simulink model "RALFMain"  (R2018b)
settings: Solver=FixedStepAuto  StartTime=0.0  StopTime=inf  FixedStep=0.001  RelTol=1e-3
InitFcn:
  | init
StopFcn:
  | stop
model workspace (MAT data in the model file):
  SL_ROS_VariableLengthArrays_MaxSizes.CommonInfo.ArrayTruncateAction = 'EmitWarning'
  SL_ROS_VariableLengthArrays_MaxSizes.MsgTypeMap = containers.Map
  SL_ROS_VariableLengthArrays_MaxSizes.MsgTypeMap.serialization.keys = {'sensor_msgs/Joy', 'std_msgs/Float32MultiArray', 'std_msgs/Int16MultiArray', 'std_msgs/Int32MultiArray', 'std_msgs/UInt16MultiArray', 'std_msgs/UInt8MultiArray'}
  SL_ROS_VariableLengthArrays_MaxSizes.MsgTypeMap.serialization.values{1}(1).PropertyName = 'Axes'
  SL_ROS_VariableLengthArrays_MaxSizes.MsgTypeMap.serialization.values{1}(1).DataType = 'single'
  SL_ROS_VariableLengthArrays_MaxSizes.MsgTypeMap.serialization.values{1}(1).MaxLength = 8
  SL_ROS_VariableLengthArrays_MaxSizes.MsgTypeMap.serialization.values{1}(2).PropertyName = 'Buttons'
  SL_ROS_VariableLengthArrays_MaxSizes.MsgTypeMap.serialization.values{1}(2).DataType = 'int32'
  SL_ROS_VariableLengthArrays_MaxSizes.MsgTypeMap.serialization.values{1}(2).MaxLength = 15
  SL_ROS_VariableLengthArrays_MaxSizes.MsgTypeMap.serialization.values{2}.PropertyName = 'Data'
  SL_ROS_VariableLengthArrays_MaxSizes.MsgTypeMap.serialization.values{2}.DataType = 'single'
  SL_ROS_VariableLengthArrays_MaxSizes.MsgTypeMap.serialization.values{2}.MaxLength = 8
  SL_ROS_VariableLengthArrays_MaxSizes.MsgTypeMap.serialization.values{3}.PropertyName = 'Data'
  SL_ROS_VariableLengthArrays_MaxSizes.MsgTypeMap.serialization.values{3}.DataType = 'int16'
  SL_ROS_VariableLengthArrays_MaxSizes.MsgTypeMap.serialization.values{3}.MaxLength = 4
  SL_ROS_VariableLengthArrays_MaxSizes.MsgTypeMap.serialization.values{4}.PropertyName = 'Data'
  SL_ROS_VariableLengthArrays_MaxSizes.MsgTypeMap.serialization.values{4}.DataType = 'int32'
  SL_ROS_VariableLengthArrays_MaxSizes.MsgTypeMap.serialization.values{4}.MaxLength = 8
  SL_ROS_VariableLengthArrays_MaxSizes.MsgTypeMap.serialization.values{5}.PropertyName = 'Data'
  SL_ROS_VariableLengthArrays_MaxSizes.MsgTypeMap.serialization.values{5}.DataType = 'uint16'
  SL_ROS_VariableLengthArrays_MaxSizes.MsgTypeMap.serialization.values{5}.MaxLength = 8
  SL_ROS_VariableLengthArrays_MaxSizes.MsgTypeMap.serialization.values{6}.PropertyName = 'Data'
  SL_ROS_VariableLengthArrays_MaxSizes.MsgTypeMap.serialization.values{6}.DataType = 'uint8'
  SL_ROS_VariableLengthArrays_MaxSizes.MsgTypeMap.serialization.values{6}.MaxLength = 8
  SL_ROS_VariableLengthArrays_MaxSizes.MsgTypeMap.serialization.uniformity = 0
  SL_ROS_VariableLengthArrays_MaxSizes.MsgTypeMap.serialization.keyType = 'char'
  SL_ROS_VariableLengthArrays_MaxSizes.MsgTypeMap.serialization.valueType = 'any'
undefined symbols (not defined in the file): Axes, Axes_SL_Info, Buttons, Buttons_SL_Info, kp, nmax, pwinkel, pwinkel_R, pwinkel_vel
libraries: simulink x15, etargetslib x10, cstblocks x4, robotlib x4, dspswit3 x4, simulink_extras x4, robotcorelib x1
CloseFcn:
  | stop
settings Model: EnablePacing=on  Creator=alf  LastModifiedBy=alf
settings OptimizationCC: EnhancedBackFolding=on  PassReuseOutputArgsAs=Individual arguments  MaxStackSize=64  OptimizeBlockOrder=speed  DifferentSizesBufferReuse=on  OptimizationCustomize=off
settings DebuggingCC: ParameterPrecisionLossMsg=none  ParameterTunabilityLossMsg=error
settings HardwareCC: ProdBitPerLong=64  ProdHWDeviceType=Intel->x86-64 (Linux 64)
settings SFSimCC: MATLABDynamicMemAlloc=off
settings RTWCC: SystemTargetFile=ert.tlc  HardwareBoard=Robot Operating System (ROS)  TLCOptions="-aInlineSetEventsForThisBaseRateFcn=TLC_FALSE -aSuppressMultiTaskScheduler=TLC_FALSE  -aRateBasedStepFcn=0"  TemplateMakefile=ert_default_tmf  GenerateReport=on  Toolchain=Catkin  IncludeHyperlinkInReport=on  LaunchReport=on  TargetLang=C++  GenerateTraceInfo=on  GenerateTraceReport=on  GenerateTraceReportSl=on  GenerateTraceReportSf=on  GenerateTraceReportEml=on
settings CodeAppCC: ForceParamTrailComments=on  IgnoreCustomStorageClasses=off  OperatorAnnotations=on  SimulinkDataObjDesc=on  SFDataObjDesc=on  InsertBlockDesc=on
settings ERTTargetCC: SupportContinuousTime=on  SupportNonInlinedSFcns=on

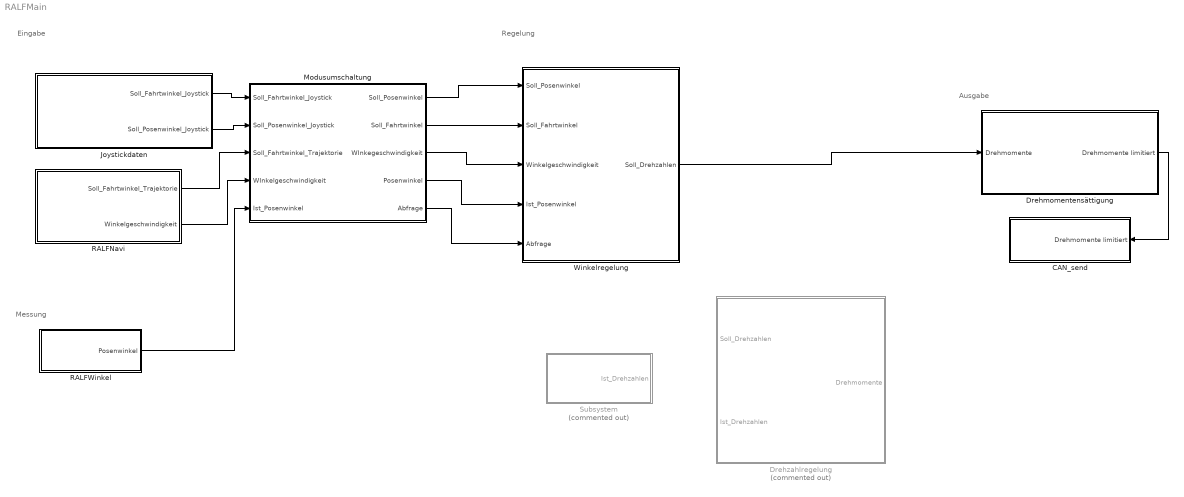
== system RALFMain ==
  note: Ausgabe
  note: Eingabe
  note: Messung
  note: Regelung
  CAN_send : Subsystem
  Drehmomentensättigung : Subsystem
  Drehzahlregelung : Subsystem  Commented=on
  Joystickdaten : Subsystem
  Modusumschaltung : Subsystem
  RALFNavi : Subsystem
  RALFWinkel : Subsystem
  Subsystem : Subsystem  Commented=on
  Winkelregelung : Subsystem
  wires:
  Modusumschaltung/1(Soll_Posenwinkel) -> Winkelregelung/1(Soll_Posenwinkel)
  Modusumschaltung/2(Soll_Fahrtwinkel) -> Winkelregelung/2(Soll_Fahrtwinkel)
  Joystickdaten/1(Soll_Fahrtwinkel_Joystick) -> Modusumschaltung/1(Soll_Fahrtwinkel_Joystick)
  Joystickdaten/2(Soll_Posenwinkel_Joystick) -> Modusumschaltung/2(Soll_Posenwinkel_Joystick)
  Modusumschaltung/4(Posenwinkel) -> Winkelregelung/4(Ist_Posenwinkel)
  Modusumschaltung/3(WInkegeschwindigkeit) -> Winkelregelung/3(Winkelgeschwindigkeit)
  RALFWinkel/1(Posenwinkel) -> Modusumschaltung/5(Ist_Posenwinkel)
  RALFNavi/1(Soll_Fahrtwinkel_Trajektorie) -> Modusumschaltung/3(Soll_Fahrtwinkel_Trajektorie)
  RALFNavi/2("Winkelgeschwindigkeit ") -> Modusumschaltung/4("WInkelgeschwindigkeit ")
  Modusumschaltung/5(Abfrage) -> Winkelregelung/5("Abfrage ")
  Drehmomentensättigung/1(Drehmomente limitiert) -> CAN_send/1(Drehmomente limitiert)
  Winkelregelung/1(Soll_Drehzahlen) -> Drehmomentensättigung/1(Drehmomente)

== system RALFMain/CAN_send ==
  Drehmomente limitiert : Inport
  CAN send back left : S-Function  FunctionName=CAN_send  Parameters=Port,Identifier  SFunctionModules=socketcan  SFunctionDeploymentMode=off  EnableBusSupport=off  mask{Port=can0, Identifier=hex2dec('121')}
      mask prompts: Port "CAN Port"
      mask TypeOptions Port: can0 | can1 | can2
      mask DialogControl DescTextVar Prompt: Dennis Hotze, Dominik Eickmann
  CAN send back right : S-Function  FunctionName=CAN_send  Parameters=Port,Identifier  SFunctionModules=socketcan  SFunctionDeploymentMode=off  EnableBusSupport=off  mask{Port=can0, Identifier=hex2dec('131')}
      mask prompts: Port "CAN Port"
      mask TypeOptions Port: can0 | can1 | can2
      mask DialogControl DescTextVar Prompt: Dennis Hotze, Dominik Eickmann
  CAN send front left : S-Function  FunctionName=CAN_send  Parameters=Port,Identifier  SFunctionModules=socketcan  SFunctionDeploymentMode=off  EnableBusSupport=off  mask{Port=can0, Identifier=hex2dec('111')}
      mask prompts: Port "CAN Port"
      mask TypeOptions Port: can0 | can1 | can2
      mask DialogControl DescTextVar Prompt: Dennis Hotze, Dominik Eickmann
  CAN send front right : S-Function  FunctionName=CAN_send  Parameters=Port,Identifier  SFunctionModules=socketcan  SFunctionDeploymentMode=off  EnableBusSupport=off  mask{Port=can0, Identifier=hex2dec('101')}
      mask prompts: Port "CAN Port"
      mask TypeOptions Port: can0 | can1 | can2
      mask DialogControl DescTextVar Prompt: Dennis Hotze, Dominik Eickmann
  Demux : Demux
  wires:
  Demux/4 -> CAN send back right/1
  Demux/1 -> CAN send front right/1
  Demux/2 -> CAN send front left/1
  Drehmomente limitiert/1 -> Demux/1
  Demux/3 -> CAN send back left/1

== system RALFMain/Drehmomentensättigung ==
  note: Inaktiv
  Drehmomente : Inport
  Abfrage DMS-Betaetigung : Subsystem
  Conversion MiControll : Subsystem
  Product : Product
  Sättigung/Conversion EPOS : Subsystem  Commented=on
  Drehmomente limitiert : Outport
  wires:
  Drehmomente/1 -> Product/1
  Abfrage DMS-Betaetigung/1("DMS-Betaetigung ") -> Product/2
  Product/1 -> Conversion MiControll/1(In1)
  Conversion MiControll/1(Out1) -> Drehmomente limitiert/1

== system RALFMain/Drehzahlregelung ==
  note: Inaktiv
  Soll_Drehzahlen : Inport
  Ist_Drehzahlen : Inport  Port=2
  PID Controller : simulink/Continuous/PID Controller  Controller=PID  Form=Ideal  TimeDomain=Continuous-time  SampleTime=-1  IntegratorMethod=Forward Euler  FilterMethod=Forward Euler  ControllerParametersSource=internal  P=0.05105  I=0.78114  D=0  UseFilter=on  N=100  TunerSelectOption=Transfer Function Based (PID Tuner App)  InitialConditionSource=internal  InitialConditionForIntegrator=0  InitialConditionForFilter=0  DifferentiatorICPrevScaledInput=0  ExternalReset=none  TrackingMode=off  Kt=1  LimitOutput=on  UpperSaturationLimit=inf  LowerSaturationLimit=-inf  LinearizeAsGain=on  AntiWindupMode=back-calculation  Kb=1  POutMin=[]  POutMax=[]  IOutMin=[]  IOutMax=[]  DOutMin=[]  DOutMax=[]  NOutMin=[]  NOutMax=[]  SumOutMin=[]  SumOutMax=[]  SaturationOutMin=[]  SaturationOutMax=[]  PParamMin=[]  PParamMax=[]  IParamMin=[]  IParamMax=[]  DParamMin=[]  DParamMax=[]  NParamMin=[]  NParamMax=[]  KbParamMin=[]  KbParamMax=[]  KtParamMin=[]  KtParamMax=[]  KbOutMin=[]  KbOutMax=[]  KtOutMin=[]  KtOutMax=[]  IntegratorOutMin=[]  IntegratorOutMax=[]  FilterOutMin=[]  FilterOutMax=[]  SumI1OutMin=[]  SumI1OutMax=[]  SumI2OutMin=[]  SumI2OutMax=[]  SumI3OutMin=[]  SumI3OutMax=[]  SumI4OutMin=[]  SumI4OutMax=[]  SumDOutMin=[]  SumDOutMax=[]  DifferentiatorOutMin=[]  DifferentiatorOutMax=[]  FilterDiffOutCoefMin=[]  FilterDiffOutCoefMax=[]  ReciprocalOutMin=[]  ReciprocalOutMax=[]  SumDenOutMin=[]  SumDenOutMax=[]  SumNumOutMin=[]  SumNumOutMax=[]  DivideOutMin=[]  DivideOutMax=[]  IntegratorContinuousStateAttributes=''  IntegratorStateMustResolveToSignalObject=off  IntegratorRTWStateStorageClass=Auto  FilterContinuousStateAttributes=''  FilterStateMustResolveToSignalObject=off  FilterRTWStateStorageClass=Auto  ParallelPVariant=Passthrough  IdealPVariant=InternalParameters  IVariant=InternalParameters  DVariant=InternalParameters  IntegratorVariant=Continuous  SatVariant=Enabled  AWVariant=BackCalculation  PCopyVariant=Disabled  TRVariant=Disabled  FdbkBlocksVariant=Forward  IdealPFdbkVariant=Disabled  SatFdbkVariant=Disabled  DerivativeFilterVariant=ContFilter  NVariant=InternalParameters  NCopyVariant=Disabled  FilterICVariant=InternalICsFilter  IntegratorICVariant=InternalICs  ExternalResetVariant=Disabled  TRSumVariant=Passthrough  SumFdbkVariant=Disabled  SumVariant=Sum_PID
  Regelung RALF : Subsystem  Commented=on
  Sum : Sum  Inputs=|+-
  Drehmomente : Outport
  wires:
  Soll_Drehzahlen/1 -> Sum/1
  Ist_Drehzahlen/1 -> Sum/2
  Sum/1 -> PID Controller/1
  PID Controller/1 -> Drehmomente/1

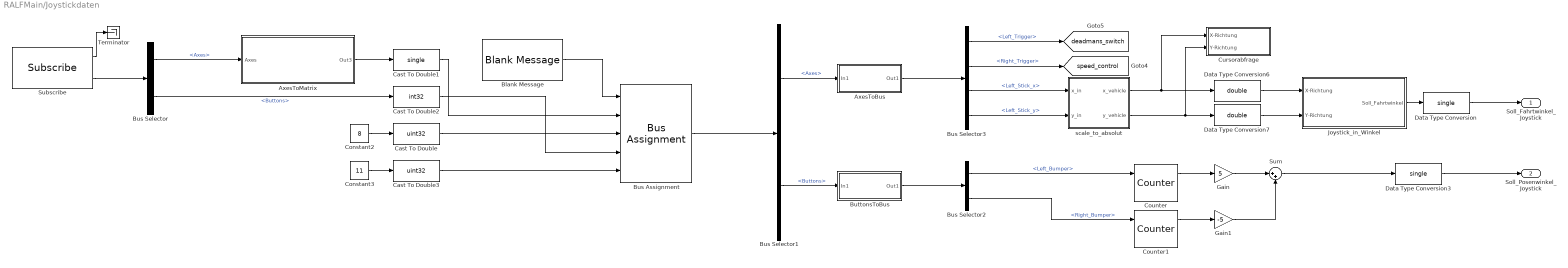
== system RALFMain/Joystickdaten ==
  AxesToBus : Subsystem
  AxesToMatrix : Subsystem
  Blank Message : robotlib/Blank Message  messageClass=Message  entityType=sensor_msgs/Joy  messageType=sensor_msgs/Joy  SampleTime=inf
      settings: SourceProductBaseCode=RO
  Bus Assignment : BusAssignment  AssignedSignals=Axes,Axes_SL_Info.CurrentLength,Buttons,Buttons_SL_Info.CurrentLength
  Bus Selector : BusSelector  OutputSignals=Axes,Buttons
  Bus Selector1 : BusSelector  OutputSignals=Axes,Buttons
  Bus Selector2 : BusSelector  OutputSignals=Bumper.Left_Bumper,Bumper.Right_Bumper
  Bus Selector3 : BusSelector  OutputSignals=Trigger.Left_Trigger,Trigger.Right_Trigger,Left_Stick.Left_Stick_x,Left_Stick.Left_Stick_y
  ButtonsToBus : Subsystem
  Cast To Double : DataTypeConversion  OutDataTypeStr=uint32
  Cast To Double1 : DataTypeConversion  OutDataTypeStr=single
  Cast To Double2 : DataTypeConversion  OutDataTypeStr=int32
  Cast To Double3 : DataTypeConversion  OutDataTypeStr=uint32
  Constant2 : Constant  Value=8
  Constant3 : Constant  Value=11
  Counter : dspswit3/Counter  Direction=Up  CountEvent=Rising edge  CounterSize=User defined  MaxCount=255  InitialCount=0  Output=Count and Hit  HitValue=32  ResetInput=on  SamplesPerFrame=1  Ts=1  CntDtype=double  HitDtype=Logical
  Counter1 : dspswit3/Counter  Direction=Up  CountEvent=Rising edge  CounterSize=User defined  MaxCount=255  InitialCount=0  Output=Count and Hit  HitValue=32  ResetInput=on  SamplesPerFrame=1  Ts=1  CntDtype=double  HitDtype=Logical
  Cursorabfrage : Subsystem
  Data Type Conversion : DataTypeConversion  OutDataTypeStr=single
  Data Type Conversion3 : DataTypeConversion  OutDataTypeStr=single
  Data Type Conversion6 : DataTypeConversion  OutDataTypeStr=double
  Data Type Conversion7 : DataTypeConversion  OutDataTypeStr=double
  Gain : Gain  Gain=5
  Gain1 : Gain  Gain=-5
  Joystick_in_Winkel : Subsystem
  Subscribe : robotlib/Subscribe  topicSource=Select from ROS network  topic=/joy  messageType=sensor_msgs/Joy  sampleTime=-1  messageQueueLength=1
      settings: SourceProductBaseCode=RO
  Sum : Sum  Inputs=|++
  Terminator : Terminator
  scale_to_absolut : Subsystem
  Soll_Fahrtwinkel_Joystick : Outport
  Soll_Posenwinkel_Joystick : Outport  Port=2
  tag scope: deadmans_switch=global, speed_control=global
  wires:
  Bus Selector2/2 -> Counter1/1  "<Right_Bumper>"
  Bus Selector2/1 -> Counter/1  "<Left_Bumper>"
  AxesToBus/1(Out1) -> Bus Selector3/1
  Bus Selector1/1 -> AxesToBus/1(In1)  "<Axes>"
  Bus Selector3/4 -> scale_to_absolut/2(y_in)  "<Left_Stick_y>"
  Bus Assignment/1 -> Bus Selector1/1
  ButtonsToBus/1(Out1) -> Bus Selector2/1
  Bus Selector3/3 -> scale_to_absolut/1(x_in)  "<Left_Stick_x>"
  Bus Selector1/2 -> ButtonsToBus/1(In1)  "<Buttons>"
  Bus Selector3/1 -> [deadmans_switch]  "<Left_Trigger>"
  scale_to_absolut/1(x_vehicle) -> Cursorabfrage/1(X-Richtung), Data Type Conversion6/1
  Data Type Conversion7/1 -> Joystick_in_Winkel/2(Y-Richtung)
  Data Type Conversion6/1 -> Joystick_in_Winkel/1(X-Richtung)
  Data Type Conversion/1 -> Soll_Fahrtwinkel_Joystick/1
  Joystick_in_Winkel/1(Soll_Fahrtwinkel) -> Data Type Conversion/1
  Data Type Conversion3/1 -> Soll_Posenwinkel_Joystick/1
  Sum/1 -> Data Type Conversion3/1
  scale_to_absolut/2(y_vehicle) -> Cursorabfrage/2(Y-Richtung), Data Type Conversion7/1
  Constant3/1 -> Cast To Double3/1
  Cast To Double1/1 -> Bus Assignment/2
  Blank Message/1 -> Bus Assignment/1
  AxesToMatrix/1(Out3) -> Cast To Double1/1
  Bus Selector/2 -> Cast To Double2/1  "<Buttons>"
  Constant2/1 -> Cast To Double/1
  Cast To Double/1 -> Bus Assignment/3
  Subscribe/2 -> Bus Selector/1
  Cast To Double2/1 -> Bus Assignment/4
  Subscribe/1 -> Terminator/1
  Bus Selector/1 -> AxesToMatrix/1(Axes)  "<Axes>"
  Cast To Double3/1 -> Bus Assignment/5
  Bus Selector3/2 -> [speed_control]  "<Right_Trigger>"
  Counter/1 -> Gain/1
  Gain/1 -> Sum/1
  Counter1/1 -> Gain1/1
  Gain1/1 -> Sum/2

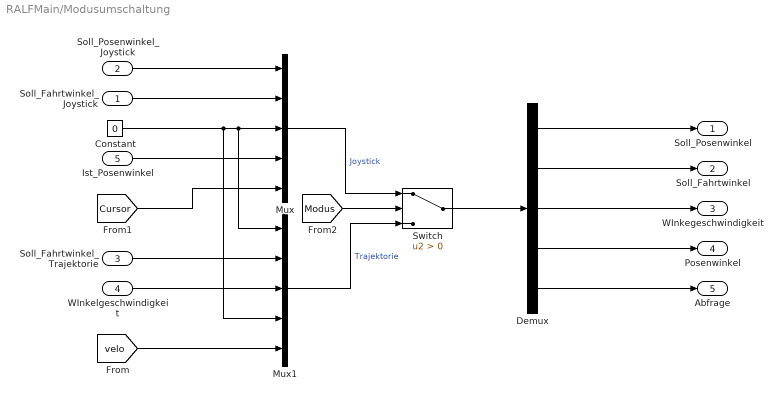
== system RALFMain/Modusumschaltung ==
  Soll_Fahrtwinkel_Joystick : Inport
  Soll_Posenwinkel_Joystick : Inport  Port=2
  Soll_Fahrtwinkel_Trajektorie : Inport  Port=3
  "WInkelgeschwindigkeit " : Inport  Port=4
  Ist_Posenwinkel : Inport  Port=5
  Constant : Constant  Value=0  OutDataTypeStr=single
  Demux : Demux  Outputs=5
  Mux : Mux  Inputs=5
  Mux1 : Mux  Inputs=5
  Switch : Switch  Criteria=u2 > Threshold
  Soll_Posenwinkel : Outport
  Soll_Fahrtwinkel : Outport  Port=2
  WInkegeschwindigkeit : Outport  Port=3
  Posenwinkel : Outport  Port=4
  Abfrage : Outport  Port=5
  wires:
  Switch/1 -> Demux/1
  Demux/2 -> Soll_Fahrtwinkel/1
  Demux/1 -> Soll_Posenwinkel/1
  Soll_Fahrtwinkel_Joystick/1 -> Mux/2
  Mux/1 -> Switch/1  "Joystick"
  Mux1/1 -> Switch/3  "Trajektorie"
  Constant/1 -> Mux1/4, Mux1/1, Mux/3
  Demux/3 -> WInkegeschwindigkeit/1
  Demux/4 -> Posenwinkel/1
  Soll_Posenwinkel_Joystick/1 -> Mux/1
  Ist_Posenwinkel/1 -> Mux/4
  Soll_Fahrtwinkel_Trajektorie/1 -> Mux1/2
  "WInkelgeschwindigkeit "/1 -> Mux1/3
  [Cursor] -> Mux/5
  [velo] -> Mux1/5
  Demux/5 -> Abfrage/1
  [Modus] -> Switch/2

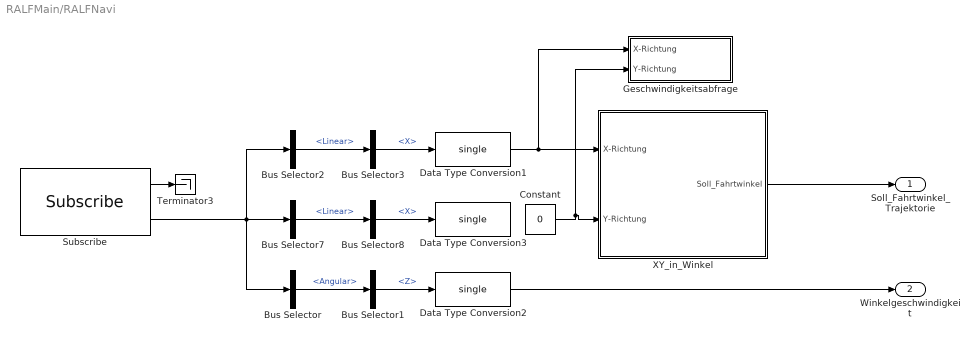
== system RALFMain/RALFNavi ==
  Bus Selector : BusSelector  OutputSignals=Angular
  Bus Selector1 : BusSelector  OutputSignals=Z
  Bus Selector2 : BusSelector  OutputSignals=Linear
  Bus Selector3 : BusSelector  OutputSignals=X
  Bus Selector7 : BusSelector  OutputSignals=Linear
  Bus Selector8 : BusSelector  OutputSignals=X
  Constant : Constant  Value=0  OutDataTypeStr=single
  Data Type Conversion1 : DataTypeConversion  OutDataTypeStr=single
  Data Type Conversion2 : DataTypeConversion  OutDataTypeStr=single
  Data Type Conversion3 : DataTypeConversion  OutDataTypeStr=single
  Geschwindigkeitsabfrage : Subsystem
  Subscribe : robotlib/Subscribe  topicSource=Select from ROS network  topic=/cmd_vel  messageType=geometry_msgs/Twist  sampleTime=-1  messageQueueLength=1
      settings: SourceProductBaseCode=RO
  Terminator3 : Terminator
  XY_in_Winkel : Subsystem
  Soll_Fahrtwinkel_Trajektorie : Outport
  "Winkelgeschwindigkeit " : Outport  Port=2
  wires:
  Bus Selector3/1 -> Data Type Conversion1/1  "<X>"
  Bus Selector2/1 -> Bus Selector3/1  "<Linear>"
  Bus Selector7/1 -> Bus Selector8/1  "<Linear>"
  Data Type Conversion2/1 -> "Winkelgeschwindigkeit "/1
  Bus Selector8/1 -> Data Type Conversion3/1  "<X>"
  Subscribe/2 -> Bus Selector7/1, Bus Selector/1, Bus Selector2/1
  Bus Selector1/1 -> Data Type Conversion2/1  "<Z>"
  Bus Selector/1 -> Bus Selector1/1  "<Angular>"
  Subscribe/1 -> Terminator3/1
  XY_in_Winkel/1(Soll_Fahrtwinkel) -> Soll_Fahrtwinkel_Trajektorie/1
  Data Type Conversion1/1 -> Geschwindigkeitsabfrage/1(X-Richtung), XY_in_Winkel/1(X-Richtung)
  Constant/1 -> Geschwindigkeitsabfrage/2(Y-Richtung), XY_in_Winkel/2(Y-Richtung)

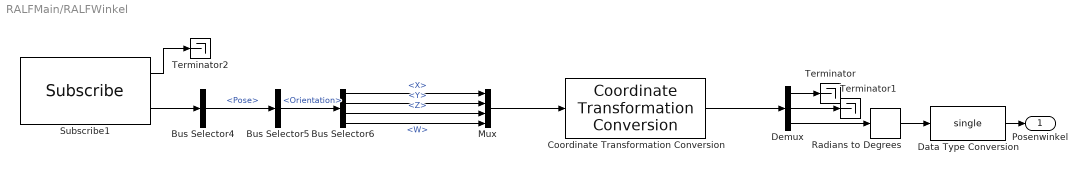
== system RALFMain/RALFWinkel ==
  Bus Selector4 : BusSelector  OutputSignals=Pose
  Bus Selector5 : BusSelector  OutputSignals=Orientation
  Bus Selector6 : BusSelector  OutputSignals=X,Y,Z,W
  Coordinate Transformation Conversion : robotcorelib/Coordinate Transformation Conversion  InputRepresentation=Quaternion  InputEulerSequence=ZYX  ShowTrVecInputPort=on  OutputRepresentation=Euler Angles  OutputEulerSequence=ZYX  ShowTrVecOutputPort=on  SimulateUsing=Interpreted execution
      settings: SourceProductBaseCode=RO
  Data Type Conversion : DataTypeConversion  OutDataTypeStr=single
  Demux : Demux  Outputs=3
  Mux : Mux
  Radians to Degrees : simulink_extras/Transformations/Radians to Degrees
  Subscribe1 : robotlib/Subscribe  topicSource=Select from ROS network  topic=/slam_out_pose  messageType=geometry_msgs/PoseStamped  sampleTime=-1  messageQueueLength=1
      settings: SourceProductBaseCode=RO
  Terminator : Terminator
  Terminator1 : Terminator
  Terminator2 : Terminator
  Posenwinkel : Outport
  wires:
  Bus Selector6/4 -> Mux/4  "<W>"
  Bus Selector6/2 -> Mux/2  "<Y>"
  Bus Selector5/1 -> Bus Selector6/1  "<Orientation>"
  Bus Selector4/1 -> Bus Selector5/1  "<Pose>"
  Mux/1 -> Coordinate Transformation Conversion/1
  Subscribe1/2 -> Bus Selector4/1
  Bus Selector6/1 -> Mux/1  "<X>"
  Bus Selector6/3 -> Mux/3  "<Z>"
  Coordinate Transformation Conversion/1 -> Demux/1
  Demux/1 -> Terminator/1
  Demux/2 -> Terminator1/1
  Demux/3 -> Radians to Degrees/1
  Subscribe1/1 -> Terminator2/1
  Radians to Degrees/1 -> Data Type Conversion/1
  Data Type Conversion/1 -> Posenwinkel/1

== system RALFMain/Subsystem ==
  note: Inaktiv
  EPOS : Subsystem  Commented=on
  MiControll : Subsystem
  Ist_Drehzahlen : Outport
  wires:
  MiControll/1(Out1) -> Ist_Drehzahlen/1

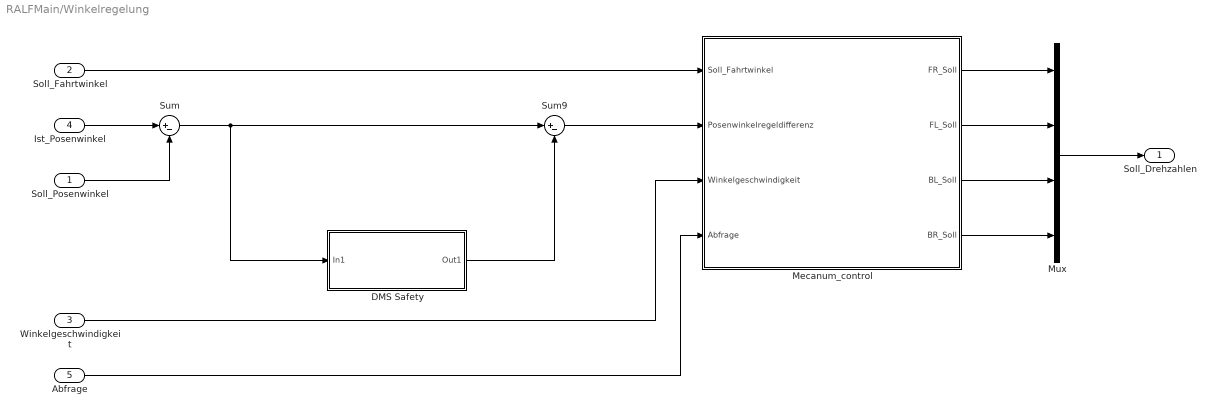
== system RALFMain/Winkelregelung ==
  Soll_Posenwinkel : Inport
  Soll_Fahrtwinkel : Inport  Port=2
  Winkelgeschwindigkeit : Inport  Port=3
  Ist_Posenwinkel : Inport  Port=4
  "Abfrage " : Inport  Port=5
  DMS Safety : Subsystem
  Mecanum_control : Subsystem
  Mux : Mux
  Sum : Sum  Inputs=|+-
  Sum9 : Sum  Inputs=|+-
  Soll_Drehzahlen : Outport
  wires:
  Soll_Posenwinkel/1 -> Sum/2
  Soll_Fahrtwinkel/1 -> Mecanum_control/1(Soll_Fahrtwinkel)
  Sum9/1 -> Mecanum_control/2(Posenwinkelregeldifferenz)
  Mecanum_control/1(FR_Soll) -> Mux/1
  Mecanum_control/4(BR_Soll) -> Mux/4
  Mecanum_control/2(FL_Soll) -> Mux/2
  Mecanum_control/3(BL_Soll) -> Mux/3
  Sum/1 -> DMS Safety/1(In1), Sum9/1
  Ist_Posenwinkel/1 -> Sum/1
  Mux/1 -> Soll_Drehzahlen/1
  Winkelgeschwindigkeit/1 -> Mecanum_control/3(Winkelgeschwindigkeit)
  "Abfrage "/1 -> Mecanum_control/4(Abfrage)
  DMS Safety/1(Out1) -> Sum9/2

== system RALFMain/Drehmomentensättigung/Abfrage DMS-Betaetigung ==
  Compare To Constant : simulink/Logic and Bit Operations/Compare To Constant  relop=>  const=0.9  OutDataTypeStr=boolean
  Data Type Conversion : DataTypeConversion  OutDataTypeStr=single
  "DMS-Betaetigung " : Outport
  wires:
  Compare To Constant/1 -> Data Type Conversion/1
  Data Type Conversion/1 -> "DMS-Betaetigung "/1
  [deadmans_switch] -> Compare To Constant/1

== system RALFMain/Drehmomentensättigung/Conversion MiControll ==
  In1 : Inport
  " " : DataTypeConversion  OutDataTypeStr=int16
  Byte Pack : etargetslib/Byte Pack  datatypes={'int16'}  byteAlign=1
  Out1 : Outport
  wires:
  " "/1 -> Byte Pack/1
  In1/1 -> " "/1
  Byte Pack/1 -> Out1/1

== system RALFMain/Drehmomentensättigung/Sättigung//Conversion EPOS ==
  In1 : Inport
  Byte Pack : etargetslib/Byte Pack  datatypes={'uint16'}  byteAlign=1
  Data Type Conversion : DataTypeConversion  OutDataTypeStr=uint16
  Saturation : Saturate  UpperLimit=100  LowerLimit=-100
  Out1 : Outport
  wires:
  Data Type Conversion/1 -> Byte Pack/1
  Saturation/1 -> Data Type Conversion/1
  In1/1 -> Saturation/1
  Byte Pack/1 -> Out1/1

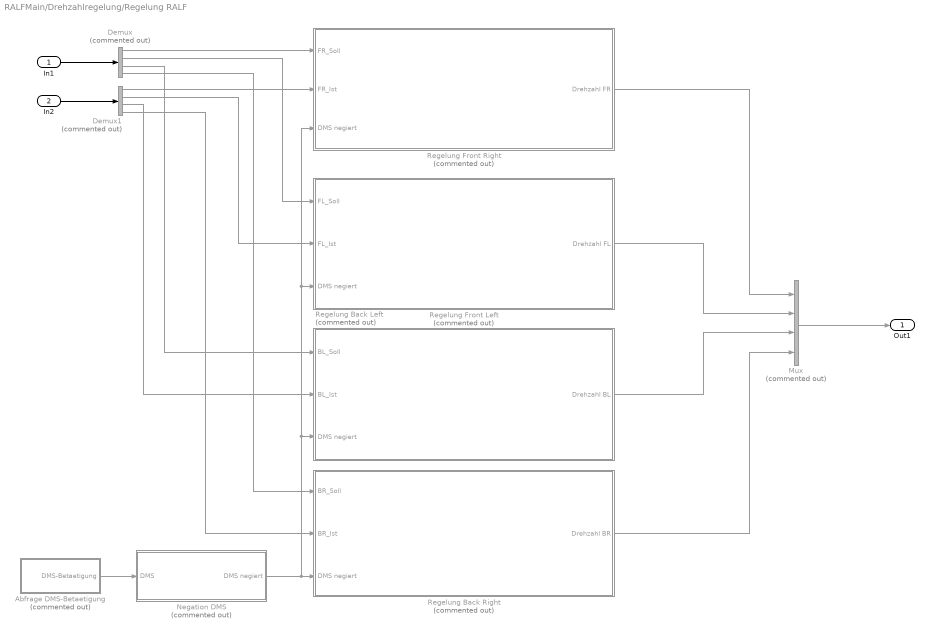
== system RALFMain/Drehzahlregelung/Regelung RALF ==
  In1 : Inport
  In2 : Inport  Port=2
  Abfrage DMS-Betaetigung : Subsystem  Commented=on
  Demux : Demux  Commented=on
  Demux1 : Demux  Commented=on
  Mux : Mux  Commented=on
  Negation DMS : Subsystem  Commented=on
  Regelung Back Left : Subsystem  Commented=on
  Regelung Back Right : Subsystem  Commented=on
  Regelung Front Left : Subsystem  Commented=on
  Regelung Front Right : Subsystem  Commented=on
  Out1 : Outport
  wires:
  Regelung Back Left/1(Drehzahl BL) -> Mux/3
  Demux/2 -> Regelung Front Left/1(FL_Soll)
  Demux/1 -> Regelung Front Right/1(FR_Soll)
  Abfrage DMS-Betaetigung/1("DMS-Betaetigung ") -> Negation DMS/1(DMS)
  Regelung Back Right/1(Drehzahl BR) -> Mux/4
  Demux1/2 -> Regelung Front Left/2(FL_Ist)
  Regelung Front Left/1(Drehzahl FL) -> Mux/2
  Regelung Front Right/1(Drehzahl FR) -> Mux/1
  Demux1/4 -> Regelung Back Right/2(BR_Ist)
  Demux/4 -> Regelung Back Right/1(BR_Soll)
  Demux/3 -> Regelung Back Left/1(BL_Soll)
  Negation DMS/1(DMS negiert) -> Regelung Back Right/3(DMS negiert), Regelung Back Left/3(DMS negiert), Regelung Front Left/3(DMS negiert), Regelung Front Right/3(DMS negiert)
  In2/1 -> Demux1/1
  In1/1 -> Demux/1
  Demux1/3 -> Regelung Back Left/2(BL_Ist)
  Demux1/1 -> Regelung Front Right/2(FR_Ist)
  Mux/1 -> Out1/1

== system RALFMain/Joystickdaten/AxesToBus ==
  In1 : Inport
  Bus Creator{4..7} (4 alike) : BusCreator  Inputs=2
  Bus Creator8 : BusCreator  Inputs=4
  Demux : Demux  Outputs=8
  Out1 : Outport
  wires:
  Bus Creator4/1 -> Bus Creator8/1  "Left_Stick"
  Bus Creator5/1 -> Bus Creator8/3  "Right_Stick"
  Bus Creator6/1 -> Bus Creator8/2  "Trigger"
  Bus Creator7/1 -> Bus Creator8/4  "Direction_Pad"
  In1/1 -> Demux/1
  Demux/1 -> Bus Creator4/1  "Left_Stick_x"
  Demux/2 -> Bus Creator4/2  "Left_Stick_y"
  Demux/4 -> Bus Creator6/2  "Right_Trigger"
  Demux/3 -> Bus Creator6/1  "Left_Trigger"
  Demux/5 -> Bus Creator5/1  "Right_Stick_x"
  Demux/6 -> Bus Creator5/2  "Right_Stick_y"
  Demux/7 -> Bus Creator7/1  "Direction_Pad_x"
  Demux/8 -> Bus Creator7/2  "Direction_Pad_y"
  Bus Creator8/1 -> Out1/1

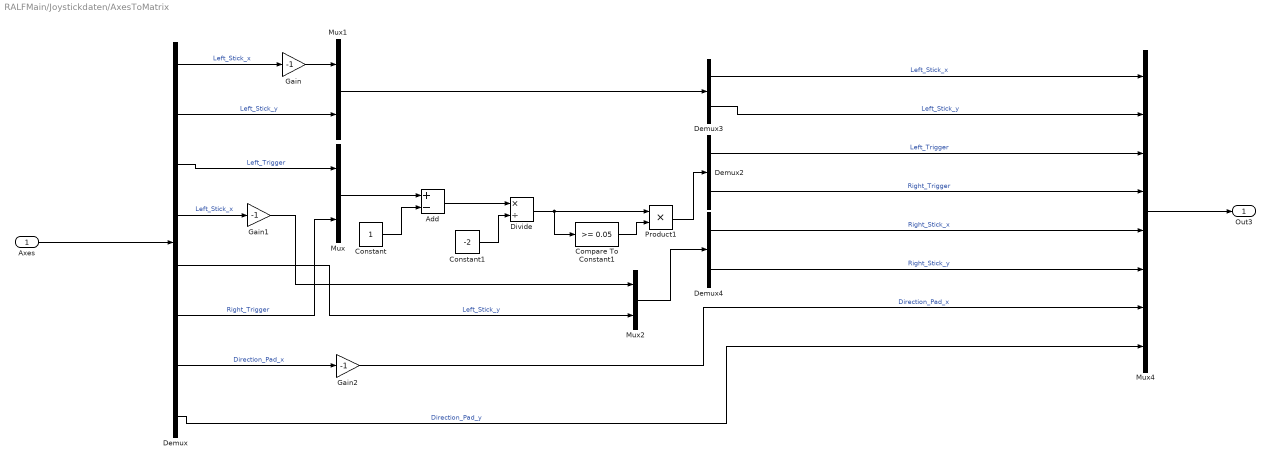
== system RALFMain/Joystickdaten/AxesToMatrix ==
  Axes : Inport
  Add : Sum  Inputs=+-
  Compare To Constant1 : simulink/Logic and Bit Operations/Compare To Constant  relop=>=  const=0.05  OutDataTypeStr=boolean
  Constant : Constant
  Constant1 : Constant  Value=-2
  Demux : Demux  Outputs=8
  Demux2 : Demux  Outputs=2
  Demux3 : Demux  Outputs=2
  Demux4 : Demux  Outputs=2
  Divide : Product  Inputs=*/
  Gain : Gain  Gain=-1
  Gain1 : Gain  Gain=-1
  Gain2 : Gain  Gain=-1
  Mux : Mux  Inputs=2
  Mux1 : Mux  Inputs=2
  Mux2 : Mux  Inputs=2
  Mux4 : Mux  Inputs=8
  Product1 : Product  OutDataTypeStr=single
  Out3 : Outport
  wires:
  Constant1/1 -> Divide/2
  Demux/5 -> Mux2/2  "Left_Stick_y"
  Demux/8 -> Mux4/8  "Direction_Pad_y"
  Mux/1 -> Add/1
  Demux/4 -> Gain1/1  "Left_Stick_x"
  Mux4/1 -> Out3/1
  Demux4/2 -> Mux4/6  "Right_Stick_y"
  Add/1 -> Divide/1
  Gain2/1 -> Mux4/7  "Direction_Pad_x"
  Demux/7 -> Gain2/1  "Direction_Pad_x"
  Demux3/1 -> Mux4/1  "Left_Stick_x"
  Demux/6 -> Mux/2  "Right_Trigger"
  Constant/1 -> Add/2
  Gain/1 -> Mux1/1
  Compare To Constant1/1 -> Product1/2
  Demux2/1 -> Mux4/3  "Left_Trigger"
  Divide/1 -> Compare To Constant1/1, Product1/1
  Product1/1 -> Demux2/1
  Demux3/2 -> Mux4/2  "Left_Stick_y"
  Demux2/2 -> Mux4/4  "Right_Trigger"
  Mux2/1 -> Demux4/1
  Demux4/1 -> Mux4/5  "Right_Stick_x"
  Axes/1 -> Demux/1
  Gain1/1 -> Mux2/1
  Demux/3 -> Mux/1  "Left_Trigger"
  Demux/1 -> Gain/1  "Left_Stick_x"
  Mux1/1 -> Demux3/1
  Demux/2 -> Mux1/2  "Left_Stick_y"

== system RALFMain/Joystickdaten/ButtonsToBus ==
  In1 : Inport
  Bus Creator : BusCreator  Inputs=6
  Bus Creator1 : BusCreator  Inputs=4
  Bus Creator2 : BusCreator  Inputs=2
  Bus Creator3 : BusCreator  Inputs=2
  Demux1 : Demux  Outputs=15
  Modusumschaltung : Subsystem
  Out1 : Outport
  wires:
  Demux1/9 -> Bus Creator/1  "XBOX_Guide_Button"
  Demux1/2 -> Modusumschaltung/1(B-Taste), Bus Creator1/2  "B"
  Demux1/11 -> Bus Creator3/2  "Right_Stick"
  Demux1/10 -> Bus Creator3/1  "Left_Stick"
  Bus Creator3/1 -> Bus Creator/6  "Sticks"
  Bus Creator1/1 -> Bus Creator/4  "ABXY"
  Demux1/1 -> Bus Creator1/1  "A"
  Bus Creator2/1 -> Bus Creator/5  "Bumper"
  Demux1/7 -> Bus Creator/3  "Back_Button"
  Demux1/4 -> Bus Creator1/4  "Y"
  Demux1/3 -> Bus Creator1/3  "X"
  Demux1/6 -> Bus Creator2/2  "Right_Bumper"
  Demux1/8 -> Bus Creator/2  "Start_Button"
  Demux1/5 -> Bus Creator2/1  "Left_Bumper"
  In1/1 -> Demux1/1
  Bus Creator/1 -> Out1/1

== system RALFMain/Joystickdaten/Cursorabfrage ==
  X-Richtung : Inport
  Y-Richtung : Inport  Port=2
  Compare To Constant : simulink/Logic and Bit Operations/Compare To Constant  relop=>=  const=0.1  OutDataTypeStr=boolean
  Compare To Constant1 : simulink/Logic and Bit Operations/Compare To Constant  relop=<=  const=-0.1  OutDataTypeStr=boolean
  Compare To Constant2 : simulink/Logic and Bit Operations/Compare To Constant  relop=<=  const=-0.1  OutDataTypeStr=boolean
  Compare To Constant3 : simulink/Logic and Bit Operations/Compare To Constant  relop=>=  const=0.1  OutDataTypeStr=boolean
  Data Type Conversion1 : DataTypeConversion  OutDataTypeStr=single
  Logical Operator1 : Logic  Operator=OR  Inputs=4  AllPortsSameDT=off  OutDataTypeStr=boolean
  tag scope: Cursor=global
  wires:
  X-Richtung/1 -> Compare To Constant1/1, Compare To Constant/1
  Y-Richtung/1 -> Compare To Constant3/1, Compare To Constant2/1
  Compare To Constant2/1 -> Logical Operator1/4
  Compare To Constant3/1 -> Logical Operator1/3
  Compare To Constant1/1 -> Logical Operator1/2
  Compare To Constant/1 -> Logical Operator1/1
  Logical Operator1/1 -> Data Type Conversion1/1
  Data Type Conversion1/1 -> [Cursor]

== system RALFMain/Joystickdaten/Joystick_in_Winkel ==
  X-Richtung : Inport
  Y-Richtung : Inport  Port=2
  Cartesian to Polar : simulink_extras/Transformations/Cartesian to Polar
      settings: SourceProductName=Simulink
  Soll_Fahrtwinkel : Outport
  wires:
  Cartesian to Polar/2 -> Soll_Fahrtwinkel/1
  X-Richtung/1 -> Cartesian to Polar/1
  Y-Richtung/1 -> Cartesian to Polar/2

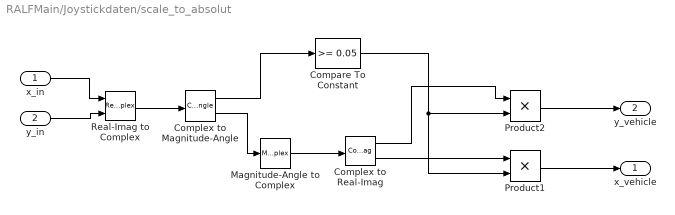
== system RALFMain/Joystickdaten/scale_to_absolut ==
  x_in : Inport
  y_in : Inport  Port=2
  Compare To Constant : simulink/Logic and Bit Operations/Compare To Constant  relop=>=  const=0.05  OutDataTypeStr=boolean
  Complex to Magnitude-Angle : ComplexToMagnitudeAngle
  Complex to Real-Imag : ComplexToRealImag
  Magnitude-Angle to Complex : MagnitudeAngleToComplex  Input=Angle  ConstantPart=1
  Product1 : Product
  Product2 : Product
  Real-Imag to Complex : RealImagToComplex
  x_vehicle : Outport
  y_vehicle : Outport  Port=2
  wires:
  Magnitude-Angle to Complex/1 -> Complex to Real-Imag/1
  Complex to Magnitude-Angle/2 -> Magnitude-Angle to Complex/1
  Product2/1 -> y_vehicle/1
  Compare To Constant/1 -> Product2/2, Product1/2
  Complex to Real-Imag/2 -> Product1/1
  Complex to Magnitude-Angle/1 -> Compare To Constant/1
  Real-Imag to Complex/1 -> Complex to Magnitude-Angle/1
  x_in/1 -> Real-Imag to Complex/1
  Complex to Real-Imag/1 -> Product2/1
  y_in/1 -> Real-Imag to Complex/2
  Product1/1 -> x_vehicle/1

== system RALFMain/RALFNavi/Geschwindigkeitsabfrage ==
  X-Richtung : Inport
  Y-Richtung : Inport  Port=2
  Compare To Constant : simulink/Logic and Bit Operations/Compare To Constant  relop=>=  const=0.1  OutDataTypeStr=boolean
  Compare To Constant1 : simulink/Logic and Bit Operations/Compare To Constant  relop=<=  const=-0.1  OutDataTypeStr=boolean
  Compare To Constant2 : simulink/Logic and Bit Operations/Compare To Constant  relop=<=  const=-0.1  OutDataTypeStr=boolean
  Compare To Constant3 : simulink/Logic and Bit Operations/Compare To Constant  relop=>=  const=0.1  OutDataTypeStr=boolean
  Data Type Conversion1 : DataTypeConversion  OutDataTypeStr=single
  Logical Operator1 : Logic  Operator=OR  Inputs=4  AllPortsSameDT=off  OutDataTypeStr=boolean
  tag scope: velo=global
  wires:
  Compare To Constant3/1 -> Logical Operator1/3
  Compare To Constant2/1 -> Logical Operator1/4
  Compare To Constant/1 -> Logical Operator1/1
  Compare To Constant1/1 -> Logical Operator1/2
  Y-Richtung/1 -> Compare To Constant3/1, Compare To Constant2/1
  X-Richtung/1 -> Compare To Constant1/1, Compare To Constant/1
  Data Type Conversion1/1 -> [velo]
  Logical Operator1/1 -> Data Type Conversion1/1

== system RALFMain/RALFNavi/XY_in_Winkel ==
  X-Richtung : Inport
  Y-Richtung : Inport  Port=2
  Cartesian to Polar : simulink_extras/Transformations/Cartesian to Polar
      settings: SourceProductName=Simulink
  Soll_Fahrtwinkel : Outport
  wires:
  Cartesian to Polar/2 -> Soll_Fahrtwinkel/1
  X-Richtung/1 -> Cartesian to Polar/1
  Y-Richtung/1 -> Cartesian to Polar/2
  Cartesian to Polar/1 -> ?

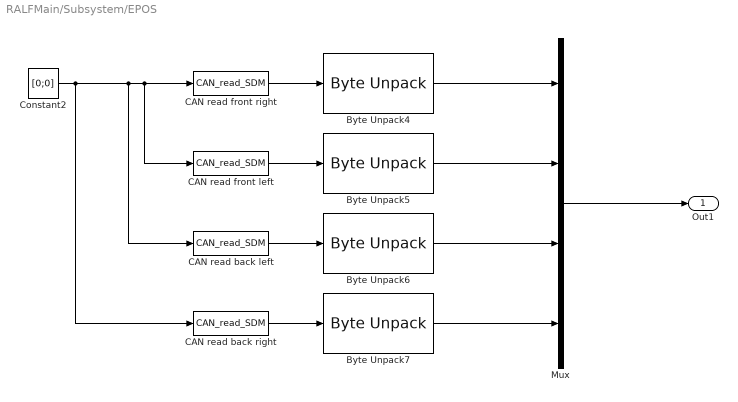
== system RALFMain/Subsystem/EPOS ==
  Byte Unpack{4..7} (4 alike) : etargetslib/Byte Unpack  dimensions={[1]}  datatypes={'int16'}  byteAlign=1
  CAN read back left : S-Function  FunctionName=CAN_read_SDM  Parameters=Port,Identifier  SFunctionModules=socketcan  SFunctionDeploymentMode=off  EnableBusSupport=off  mask{Port=can0, Identifier=hex2dec('123')}
      mask prompts: Port "CAN Port"
      mask TypeOptions Port: can0 | can1 | can2
      mask DialogControl DescTextVar Prompt: Dennis Hotze, Dominik Eickmann
  CAN read back right : S-Function  FunctionName=CAN_read_SDM  Parameters=Port,Identifier  SFunctionModules=socketcan  SFunctionDeploymentMode=off  EnableBusSupport=off  mask{Port=can0, Identifier=hex2dec('133')}
      mask prompts: Port "CAN Port"
      mask TypeOptions Port: can0 | can1 | can2
      mask DialogControl DescTextVar Prompt: Dennis Hotze, Dominik Eickmann
  CAN read front left : S-Function  FunctionName=CAN_read_SDM  Parameters=Port,Identifier  SFunctionModules=socketcan  SFunctionDeploymentMode=off  EnableBusSupport=off  mask{Port=can0, Identifier=hex2dec('113')}
      mask prompts: Port "CAN Port"
      mask TypeOptions Port: can0 | can1 | can2
      mask DialogControl DescTextVar Prompt: Dennis Hotze, Dominik Eickmann
  "CAN read front right " : S-Function  FunctionName=CAN_read_SDM  Parameters=Port,Identifier  SFunctionModules=socketcan  SFunctionDeploymentMode=off  EnableBusSupport=off  mask{Port=can0, Identifier=hex2dec('103')}
      mask prompts: Port "CAN Port"
      mask TypeOptions Port: can0 | can1 | can2
      mask DialogControl DescTextVar Prompt: Dennis Hotze, Dominik Eickmann
  Constant2 : Constant  Value=[0;0]
  Mux : Mux
  Out1 : Outport
  wires:
  Byte Unpack7/1 -> Mux/4
  "CAN read front right "/1 -> Byte Unpack4/1
  Byte Unpack6/1 -> Mux/3
  CAN read back right/1 -> Byte Unpack7/1
  CAN read back left/1 -> Byte Unpack6/1
  CAN read front left/1 -> Byte Unpack5/1
  Mux/1 -> Out1/1
  Constant2/1 -> CAN read back left/1, CAN read front left/1, "CAN read front right "/1, CAN read back right/1
  Byte Unpack4/1 -> Mux/1
  Byte Unpack5/1 -> Mux/2

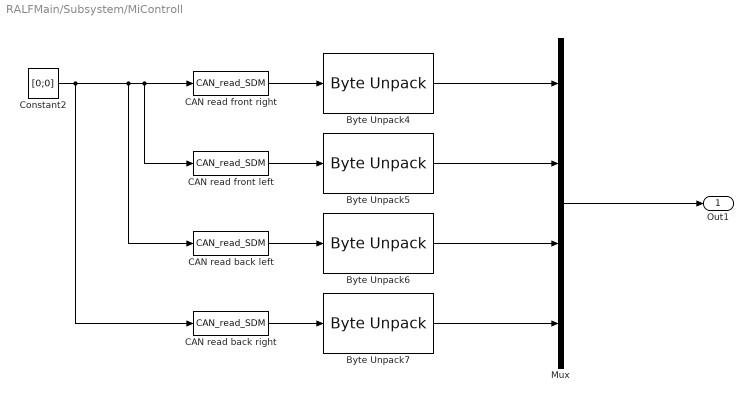
== system RALFMain/Subsystem/MiControll ==
  Byte Unpack{4..7} (4 alike) : etargetslib/Byte Unpack  dimensions={[1]}  datatypes={'int16'}  byteAlign=1
  CAN read back left : S-Function  FunctionName=CAN_read_SDM  Parameters=Port,Identifier  SFunctionModules=socketcan  SFunctionDeploymentMode=off  EnableBusSupport=off  mask{Port=can0, Identifier=hex2dec('123')}
      mask prompts: Port "CAN Port"
      mask TypeOptions Port: can0 | can1 | can2
      mask DialogControl DescTextVar Prompt: Dennis Hotze, Dominik Eickmann
  CAN read back right : S-Function  FunctionName=CAN_read_SDM  Parameters=Port,Identifier  SFunctionModules=socketcan  SFunctionDeploymentMode=off  EnableBusSupport=off  mask{Port=can0, Identifier=hex2dec('133')}
      mask prompts: Port "CAN Port"
      mask TypeOptions Port: can0 | can1 | can2
      mask DialogControl DescTextVar Prompt: Dennis Hotze, Dominik Eickmann
  CAN read front left : S-Function  FunctionName=CAN_read_SDM  Parameters=Port,Identifier  SFunctionModules=socketcan  SFunctionDeploymentMode=off  EnableBusSupport=off  mask{Port=can0, Identifier=hex2dec('113')}
      mask prompts: Port "CAN Port"
      mask TypeOptions Port: can0 | can1 | can2
      mask DialogControl DescTextVar Prompt: Dennis Hotze, Dominik Eickmann
  "CAN read front right " : S-Function  FunctionName=CAN_read_SDM  Parameters=Port,Identifier  SFunctionModules=socketcan  SFunctionDeploymentMode=off  EnableBusSupport=off  mask{Port=can0, Identifier=hex2dec('103')}
      mask prompts: Port "CAN Port"
      mask TypeOptions Port: can0 | can1 | can2
      mask DialogControl DescTextVar Prompt: Dennis Hotze, Dominik Eickmann
  Constant2 : Constant  Value=[0;0]
  Mux : Mux
  Out1 : Outport
  wires:
  Mux/1 -> Out1/1
  CAN read back left/1 -> Byte Unpack6/1
  CAN read front left/1 -> Byte Unpack5/1
  Constant2/1 -> CAN read back left/1, CAN read front left/1, "CAN read front right "/1, CAN read back right/1
  CAN read back right/1 -> Byte Unpack7/1
  Byte Unpack7/1 -> Mux/4
  Byte Unpack6/1 -> Mux/3
  Byte Unpack5/1 -> Mux/2
  "CAN read front right "/1 -> Byte Unpack4/1
  Byte Unpack4/1 -> Mux/1

== system RALFMain/Winkelregelung/DMS Safety ==
  In1 : Inport
  Abfrage DMS-Betaetigung : Subsystem
  Data Type Conversion : DataTypeConversion  OutDataTypeStr=single
  If Action Subsystem : Subsystem  TreatAsAtomicUnit=on
  Negation DMS : Subsystem
  Switch Case : SwitchCase
  Out1 : Outport
  wires:
  Negation DMS/1(DMS negiert) -> Data Type Conversion/1
  Data Type Conversion/1 -> Switch Case/1
  Switch Case/1 -> If Action Subsystem/Action
  In1/1 -> If Action Subsystem/1(In1)
  If Action Subsystem/1(Out1) -> Out1/1
  Abfrage DMS-Betaetigung/1("DMS-Betaetigung ") -> Negation DMS/1(DMS)

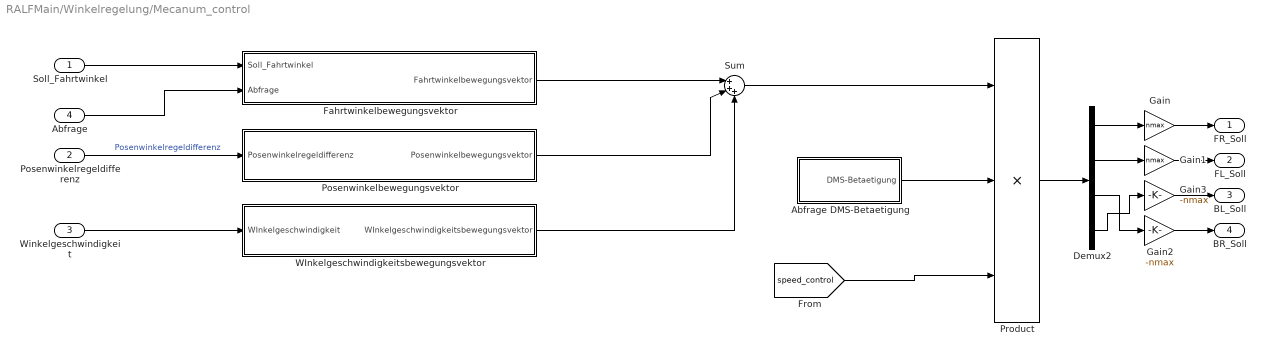
== system RALFMain/Winkelregelung/Mecanum_control ==
  Soll_Fahrtwinkel : Inport  OutDataTypeStr=single
  Posenwinkelregeldifferenz : Inport  Port=2  OutDataTypeStr=single
  Winkelgeschwindigkeit : Inport  Port=3  OutDataTypeStr=single
  Abfrage : Inport  Port=4  OutDataTypeStr=single
  Abfrage DMS-Betaetigung : Subsystem
  Demux2 : Demux
  Fahrtwinkelbewegungsvektor : Subsystem
  Gain : Gain  Gain=nmax  OutDataTypeStr=double
  Gain1 : Gain  Gain=nmax  OutDataTypeStr=double
  Gain2 : Gain  Gain=-nmax  OutDataTypeStr=double
  Gain3 : Gain  Gain=-nmax  OutDataTypeStr=double
  Posenwinkelbewegungsvektor : Subsystem
  Product : Product  Inputs=3  OutDataTypeStr=single
  Sum : Sum  Inputs=|+++
  WInkelgeschwindigkeitsbewegungsvektor : Subsystem
  FR_Soll : Outport
  FL_Soll : Outport  Port=2
  BL_Soll : Outport  Port=3
  BR_Soll : Outport  Port=4
  wires:
  Product/1 -> Demux2/1
  Demux2/2 -> Gain1/1
  Demux2/1 -> Gain/1
  Gain3/1 -> BL_Soll/1
  Gain2/1 -> BR_Soll/1
  Gain1/1 -> FL_Soll/1
  Gain/1 -> FR_Soll/1
  Demux2/3 -> Gain2/1
  Demux2/4 -> Gain3/1
  Fahrtwinkelbewegungsvektor/1(Fahrtwinkelbewegungsvektor) -> Sum/1
  Sum/1 -> Product/1
  Posenwinkelregeldifferenz/1 -> Posenwinkelbewegungsvektor/1(Posenwinkelregeldifferenz)  "Posenwinkelregeldifferenz"
  Posenwinkelbewegungsvektor/1("Posenwinkelbewegungsvektor ") -> Sum/2
  Soll_Fahrtwinkel/1 -> Fahrtwinkelbewegungsvektor/1(Soll_Fahrtwinkel)
  Winkelgeschwindigkeit/1 -> WInkelgeschwindigkeitsbewegungsvektor/1(WInkelgeschwindigkeit)
  WInkelgeschwindigkeitsbewegungsvektor/1("WInkelgeschwindigkeitsbewegungsvektor ") -> Sum/3
  Abfrage/1 -> Fahrtwinkelbewegungsvektor/2(Abfrage)
  Abfrage DMS-Betaetigung/1("DMS-Betaetigung ") -> Product/2
  [speed_control] -> Product/3

== system RALFMain/Drehzahlregelung/Regelung RALF/Abfrage DMS-Betaetigung ==
  Compare To Constant : simulink/Logic and Bit Operations/Compare To Constant  relop=>  const=0.9  OutDataTypeStr=boolean
  Data Type Conversion : DataTypeConversion  OutDataTypeStr=single
  "DMS-Betaetigung " : Outport
  wires:
  Compare To Constant/1 -> Data Type Conversion/1
  Data Type Conversion/1 -> "DMS-Betaetigung "/1
  [deadmans_switch] -> Compare To Constant/1

== system RALFMain/Drehzahlregelung/Regelung RALF/Negation DMS ==
  DMS : Inport
  Constant : Constant  Value=-1
  Product1 : Product
  Sum4 : Sum  Inputs=|++
  DMS negiert : Outport
  wires:
  DMS/1 -> Sum4/1
  Constant/1 -> Product1/2, Sum4/2
  Sum4/1 -> Product1/1
  Product1/1 -> DMS negiert/1

== system RALFMain/Drehzahlregelung/Regelung RALF/Regelung Back Left ==
  BL_Soll : Inport
  BL_Ist : Inport  Port=2
  DMS negiert : Inport  Port=3
  Constant : Constant  Value=pwinkel_R
  Gain3 : Gain  Gain=kp
  LTI System3 : cstblocks/LTI System  sys=gpidv  IC=[]
  Product4 : Product  Inputs=3
  Sum : Sum  Inputs=|+-
  Sum6 : Sum  Inputs=|+-
  Drehzahl BL : Outport
  wires:
  Sum/1 -> Sum6/1
  Gain3/1 -> Drehzahl BL/1
  BL_Ist/1 -> Sum/2
  Constant/1 -> Product4/3
  DMS negiert/1 -> Product4/2
  Product4/1 -> Sum6/2
  Sum6/1 -> LTI System3/1
  BL_Soll/1 -> Sum/1
  LTI System3/1 -> Product4/1, Gain3/1

== system RALFMain/Drehzahlregelung/Regelung RALF/Regelung Back Right ==
  BR_Soll : Inport
  BR_Ist : Inport  Port=2
  DMS negiert : Inport  Port=3
  Constant : Constant  Value=pwinkel_R
  Gain3 : Gain  Gain=kp
  LTI System3 : cstblocks/LTI System  sys=gpidv  IC=[]
  Product4 : Product  Inputs=3
  Sum : Sum  Inputs=|+-
  Sum6 : Sum  Inputs=|+-
  Drehzahl BR : Outport
  wires:
  LTI System3/1 -> Product4/1, Gain3/1
  Sum/1 -> Sum6/1
  Gain3/1 -> Drehzahl BR/1
  Constant/1 -> Product4/3
  BR_Ist/1 -> Sum/2
  DMS negiert/1 -> Product4/2
  Sum6/1 -> LTI System3/1
  Product4/1 -> Sum6/2
  BR_Soll/1 -> Sum/1

== system RALFMain/Drehzahlregelung/Regelung RALF/Regelung Front Left ==
  FL_Soll : Inport
  FL_Ist : Inport  Port=2
  DMS negiert : Inport  Port=3
  Constant : Constant  Value=pwinkel_R
  Gain3 : Gain  Gain=kp
  LTI System3 : cstblocks/LTI System  sys=gpidv  IC=[]
  Product4 : Product  Inputs=3
  Sum : Sum  Inputs=|+-
  Sum6 : Sum  Inputs=|+-
  Drehzahl FL : Outport
  wires:
  Sum/1 -> Sum6/1
  Gain3/1 -> Drehzahl FL/1
  FL_Ist/1 -> Sum/2
  Constant/1 -> Product4/3
  DMS negiert/1 -> Product4/2
  Product4/1 -> Sum6/2
  Sum6/1 -> LTI System3/1
  FL_Soll/1 -> Sum/1
  LTI System3/1 -> Product4/1, Gain3/1

== system RALFMain/Drehzahlregelung/Regelung RALF/Regelung Front Right ==
  FR_Soll : Inport
  FR_Ist : Inport  Port=2
  DMS negiert : Inport  Port=3
  Constant : Constant  Value=pwinkel_R
  Gain3 : Gain  Gain=kp
  LTI System3 : cstblocks/LTI System  sys=gpidv  IC=[]
  Product4 : Product  Inputs=3
  Sum : Sum  Inputs=|+-
  Sum6 : Sum  Inputs=|+-
  Drehzahl FR : Outport
  wires:
  Gain3/1 -> Drehzahl FR/1
  LTI System3/1 -> Product4/1, Gain3/1
  Sum/1 -> Sum6/1
  FR_Ist/1 -> Sum/2
  Sum6/1 -> LTI System3/1
  FR_Soll/1 -> Sum/1
  Product4/1 -> Sum6/2
  Constant/1 -> Product4/3
  DMS negiert/1 -> Product4/2

== system RALFMain/Joystickdaten/ButtonsToBus/Modusumschaltung ==
  B-Taste : Inport
  Constant : Constant  Value=2  OutDataTypeStr=single
  Counter : dspswit3/Counter  Direction=Up  CountEvent=Rising edge  CounterSize=User defined  MaxCount=255  InitialCount=0  Output=Count and Hit  HitValue=32  ResetInput=on  SamplesPerFrame=1  Ts=1  CntDtype=double  HitDtype=Logical
  Data Type Conversion : DataTypeConversion  OutDataTypeStr=single
  Data Type Conversion1 : DataTypeConversion  OutDataTypeStr=single
  Edge Detector : dspswit3/Edge Detector  InputProcessing=Columns as channels (frame based)
      settings: SourceProductName=DSP System Toolbox  SourceProductBaseCode=DS
  Math Function : Math  Operator=mod  SaturateOnIntegerOverflow=on
  tag scope: Modus=global
  wires:
  B-Taste/1 -> Data Type Conversion/1
  Data Type Conversion1/1 -> Math Function/1
  Edge Detector/1 -> Counter/1
  Data Type Conversion/1 -> Edge Detector/1
  Constant/1 -> Math Function/2
  Counter/1 -> Data Type Conversion1/1
  Math Function/1 -> [Modus]

== system RALFMain/Winkelregelung/DMS Safety/Abfrage DMS-Betaetigung ==
  Compare To Constant : simulink/Logic and Bit Operations/Compare To Constant  relop=>  const=0.9  OutDataTypeStr=boolean
  Data Type Conversion : DataTypeConversion  OutDataTypeStr=single
  "DMS-Betaetigung " : Outport
  wires:
  Compare To Constant/1 -> Data Type Conversion/1
  Data Type Conversion/1 -> "DMS-Betaetigung "/1
  [deadmans_switch] -> Compare To Constant/1

== system RALFMain/Winkelregelung/DMS Safety/If Action Subsystem ==
  In1 : Inport
  Action Port : ActionPort  ActionType=case
  Out1 : Outport
  wires:
  In1/1 -> Out1/1

== system RALFMain/Winkelregelung/DMS Safety/Negation DMS ==
  DMS : Inport
  Constant : Constant  Value=-1
  Product1 : Product
  Sum4 : Sum  Inputs=|++
  DMS negiert : Outport
  wires:
  DMS/1 -> Sum4/1
  Constant/1 -> Product1/2, Sum4/2
  Sum4/1 -> Product1/1
  Product1/1 -> DMS negiert/1

== system RALFMain/Winkelregelung/Mecanum_control/Abfrage DMS-Betaetigung ==
  Compare To Constant : simulink/Logic and Bit Operations/Compare To Constant  relop=>  const=0.9  OutDataTypeStr=boolean
  Data Type Conversion : DataTypeConversion  OutDataTypeStr=single
  "DMS-Betaetigung " : Outport
  wires:
  Compare To Constant/1 -> Data Type Conversion/1
  Data Type Conversion/1 -> "DMS-Betaetigung "/1
  [deadmans_switch] -> Compare To Constant/1

== system RALFMain/Winkelregelung/Mecanum_control/Fahrtwinkelbewegungsvektor ==
  Soll_Fahrtwinkel : Inport
  Abfrage : Inport  Port=2
  Constant : Constant  Value=[1 -1;1 1;1 1;1 -1]  OutDataTypeStr=single
  Mux1 : Mux  Inputs=2
  Polar to Cartesian : simulink_extras/Transformations/Polar to Cartesian
      settings: SourceProductName=Simulink  SourceProductBaseCode=SL
  Product1 : Product  Multiplication=Matrix(*)
  Saturation3 : Saturate  UpperLimit=1  LowerLimit=-1
  Fahrtwinkelbewegungsvektor : Outport
  wires:
  Soll_Fahrtwinkel/1 -> Polar to Cartesian/2
  Polar to Cartesian/2 -> Mux1/2
  Constant/1 -> Product1/1
  Product1/1 -> Saturation3/1
  Abfrage/1 -> Polar to Cartesian/1
  Polar to Cartesian/1 -> Mux1/1
  Mux1/1 -> Product1/2
  Saturation3/1 -> Fahrtwinkelbewegungsvektor/1

== system RALFMain/Winkelregelung/Mecanum_control/Posenwinkelbewegungsvektor ==
  Posenwinkelregeldifferenz : Inport
  Constant1 : Constant  Value=[-1;1;-1;1]  OutDataTypeStr=single
  Gain4 : Gain  Gain=pwinkel
  Product2 : Product  Multiplication=Matrix(*)
  "Posenwinkelbewegungsvektor " : Outport
  wires:
  Constant1/1 -> Product2/1
  Gain4/1 -> Product2/2
  Product2/1 -> "Posenwinkelbewegungsvektor "/1
  Posenwinkelregeldifferenz/1 -> Gain4/1

== system RALFMain/Winkelregelung/Mecanum_control/WInkelgeschwindigkeitsbewegungsvektor ==
  WInkelgeschwindigkeit : Inport
  Constant1 : Constant  Value=[-1;1;-1;1]  OutDataTypeStr=single
  Gain4 : Gain  Gain=pwinkel_vel
  Product2 : Product  Multiplication=Matrix(*)
  "WInkelgeschwindigkeitsbewegungsvektor " : Outport
  wires:
  Constant1/1 -> Product2/1
  Gain4/1 -> Product2/2
  Product2/1 -> "WInkelgeschwindigkeitsbewegungsvektor "/1
  WInkelgeschwindigkeit/1 -> Gain4/1
